simulink subsystem "ControlObject"  (R2023a)
settings: Solver=VariableStepAuto  StartTime=0.0  StopTime=10.0  RelTol=1e-3
settings Model: Creator=lehas  LastModifiedBy=lehas

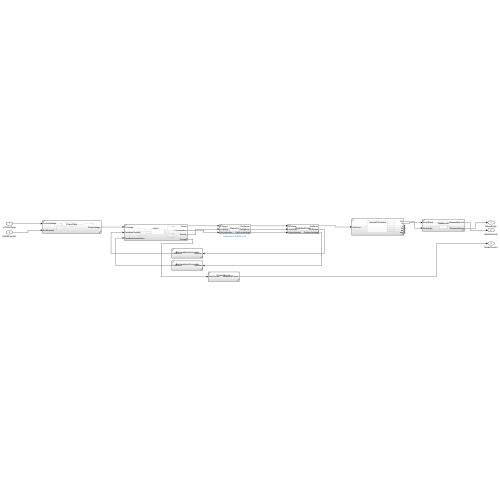
[thumbnail: Simulink's stored preview of the top-level diagram]
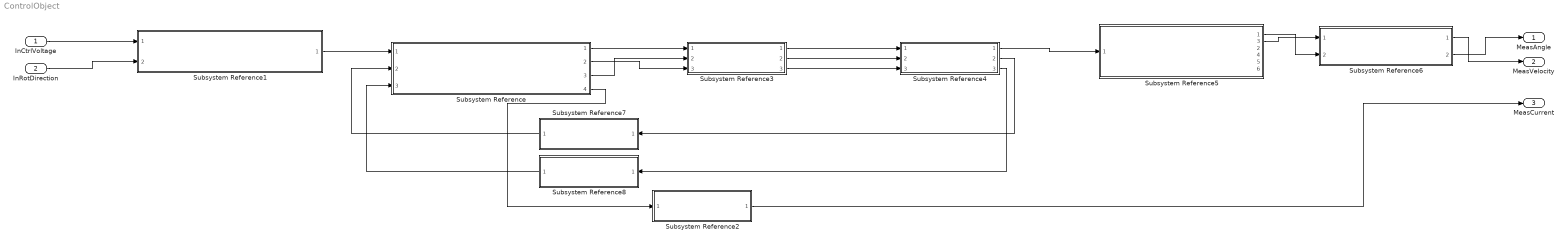
== system ControlObject ==
  InCtrlVoltage : Inport
  InRotDirection : Inport  Port=2
  Subsystem Reference : Subsystem  ReferencedSubsystem=motor
  Subsystem Reference1 : Subsystem  ReferencedSubsystem=PowerGain
  Subsystem Reference2 : Subsystem  ReferencedSubsystem=CurrentSensor
  Subsystem Reference3 : Subsystem  ReferencedSubsystem=Reductor
  Subsystem Reference4 : Subsystem  ReferencedSubsystem=RackAndPinion
  Subsystem Reference5 : Subsystem  ReferencedSubsystem=InversePendulum
      settings: PortSchema="{\"entries\":[{\"content\":{\"sides\":[{\"content\":{\"connectorIds\":[\"In1\"]},\"type\":\"ConnectorPlacement.EquallySpacedRectSide\",\"uuid\":\"6c268b52-f2b0-4a63-8568-2a842c093f71\"},{\"content\":{\"connectorIds\":[\"Out1\",\"Out3\",\"Out2\",\"Out4\",\"Out5\",\"Out6\"],\"side\":\"RIGHT\"},\"type\":\"ConnectorPlacement.EquallySpacedRectSide\",\"uuid\":\"45f7ad73-0d54-46cb-bed8-b89b6e4a225c\"},{\"content\":{\"side\":\"TOP\"},\"type\":\"ConnectorPlacement.EquallySpacedRectSide\",\"uuid\":\"e3d6e675-7829-4c15-93ec-a08051042e02\"}]},\"type\":\"ConnectorPlacement.EquallySpacedConnector\",\"uuid\":\"f5cc6c2b-eb8a-4675-b408-a4abc6a8d625\"}],\"packageUris\":[\"http://schema.mathworks.com/mf0/Connector/R2020b\"],\"version\":\"1.0\"}"
  Subsystem Reference6 : Subsystem  ReferencedSubsystem=HallSensor
  Subsystem Reference7 : Subsystem  ReferencedSubsystem=BackwardAccConverter
  Subsystem Reference8 : Subsystem  ReferencedSubsystem=BackwardAccConverter
  MeasAngle : Outport
  MeasVelocity : Outport  Port=2
  MeasCurrent : Outport  Port=3
  wires:
  InCtrlVoltage/1 -> Subsystem Reference1/1
  InRotDirection/1 -> Subsystem Reference1/2
  Subsystem Reference1/1 -> Subsystem Reference/1
  Subsystem Reference/4 -> Subsystem Reference2/1
  Subsystem Reference2/1 -> MeasCurrent/1
  Subsystem Reference/1 -> Subsystem Reference3/1
  Subsystem Reference/2 -> Subsystem Reference3/3
  Subsystem Reference/3 -> Subsystem Reference3/2
  Subsystem Reference3/1 -> Subsystem Reference4/1
  Subsystem Reference3/2 -> Subsystem Reference4/2
  Subsystem Reference3/3 -> Subsystem Reference4/3
  Subsystem Reference4/1 -> Subsystem Reference5/1
  Subsystem Reference4/2 -> Subsystem Reference7/1
  Subsystem Reference7/1 -> Subsystem Reference/2
  Subsystem Reference4/3 -> Subsystem Reference8/1
  Subsystem Reference8/1 -> Subsystem Reference/3
  Subsystem Reference5/1 -> Subsystem Reference6/2
  Subsystem Reference6/2 -> MeasAngle/1
  Subsystem Reference6/1 -> MeasVelocity/1
  Subsystem Reference5/3 -> Subsystem Reference6/1
